simulink model "Tire_Force_Observer_2016a"  (R2016a)
settings: Solver=VariableStepAuto  SolverMode=SingleTasking  StartTime=0.0  StopTime=10.0  RelTol=1e-3
undefined symbols (not defined in the file): A, B, C, DiscIntNeverNeededParam, K, TFO_Ts
settings Model: Creator=univ4123  LastModifiedBy=univ4123
settings DebuggingCC: SFUnexpectedBacktrackingDiag=error  SFNoUnconditionalDefaultTransitionDiag=error
settings SFSimCC: SimUseLocalCustomCode=on
settings RTWCC: RTWUseLocalCustomCode=on
settings GRTTargetCC: TargetLangStandard=C99 (ISO)  GeneratePreprocessorConditionals=Use local settings
settings ConfigComp: CovMetricSettings=dwe  CovHtmlReporting=off  CovSaveCumulativeToWorkspaceVar=off  CovSaveSingleToWorkspaceVar=off  CovExternalEMLEnable=on

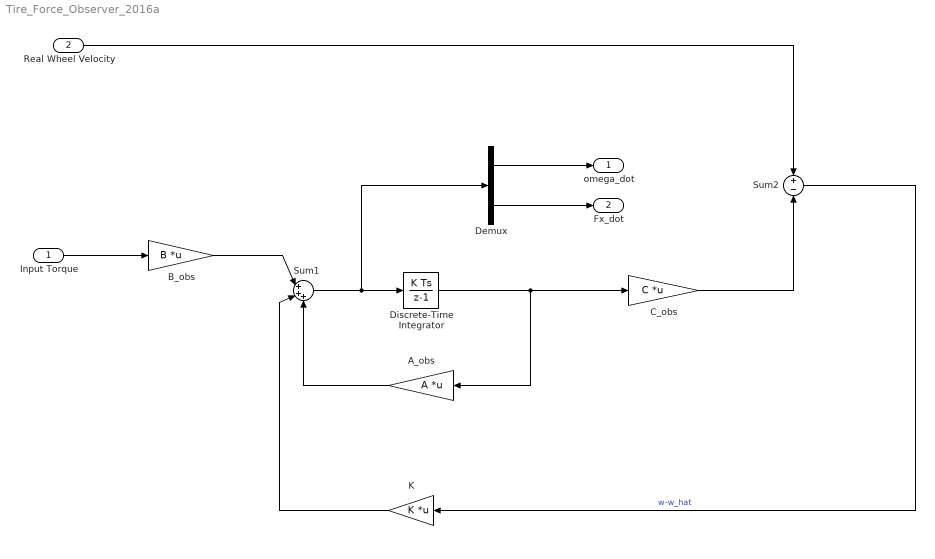
== system Tire_Force_Observer_2016a ==
  Input Torque : Inport
  Real Wheel Velocity : Inport  Port=2
  A_obs : Gain  Gain=A  Multiplication=Matrix(K*u) (u vector)
  B_obs : Gain  Gain=B  Multiplication=Matrix(K*u) (u vector)
  C_obs : Gain  Gain=C  Multiplication=Matrix(K*u) (u vector)
  Demux : Demux  Outputs=2
  Discrete-Time Integrator : DiscreteIntegrator  InitialConditionSetting=State (most efficient)  SampleTime=TFO_Ts  ICPrevOutput=DiscIntNeverNeededParam  ICPrevScaledInput=DiscIntNeverNeededParam
  K : Gain  Gain=K  Multiplication=Matrix(K*u)
  Sum1 : Sum  Inputs=|+++
  Sum2 : Sum  Inputs=+|-
  "omega_dot " : Outport
  Fx_dot : Outport  Port=2
  wires:
  Demux/2 -> Fx_dot/1
  Demux/1 -> "omega_dot "/1
  A_obs/1 -> Sum1/3
  K/1 -> Sum1/2
  C_obs/1 -> Sum2/2
  B_obs/1 -> Sum1/1
  Sum2/1 -> K/1  "w-w_hat"
  Discrete-Time Integrator/1 -> A_obs/1, C_obs/1
  Sum1/1 -> Discrete-Time Integrator/1, Demux/1
  Input Torque/1 -> B_obs/1
  Real Wheel Velocity/1 -> Sum2/1
